simulink model "AC_DER_basic_model"  (R2021b)
settings: Solver=ode3  StartTime=0.0  StopTime=0.1  FixedStep=Ts  MaxStep=0.001  RelTol=1e-3  EnableMultiTasking=on
PostLoadFcn:
  | Ts=100e-6;
InitFcn:
  | Ts=100e-6;
libraries: fl_lib x5, nesl_utility x5, opal_lib x3, rtlab x2, ee_lib x2, spsRMSLib x2
Description:
  | Full-Wave Bridge Rectifier
  | 
  | This is a model of a power supply that converts 120 volts AC to 12  volts DC. The
  | transformer has a turns ratio of 14, stepping the supply down to 8.6 volts rms, i.e.
  | 8.6*sqrt(2) = 12 volts pk-pk. The full-wave bridge rectifier plus capacitor combination
  | then converts this to DC. The resistor represents a typical load.
  | 
  | The model can be used to size the capacitor required for a specified load.  For a
  | given size of capacitor, as the load resistance is increased, the ripple on the DC
  | voltage increases. The model can also be used to drive an application circuit in
  | order to assess the effect of the ripple.
  | 
  | 
  | Copyright 2008 The MathWorks(TM), Inc.
settings Model: Creator=rhyde  LastModifiedBy=fghow
settings SolverCC: AlgebraicLoopSolver=TrustRegion
settings DataIOCC: LimitDataPoints=on  SaveFormat=Array  SignalLoggingSaveFormat=ModelDataLogs  SaveOutput=off  SignalLogging=off  SaveTime=off  ReturnWorkspaceOutputs=off
settings OptimizationCC: BlockReduction=off  OptimizeBlockIOStorage=off  BufferReuse=off  ExpressionFolding=off  ExpressionDepthLimit=2147483647  LocalBlockOutputs=off  InitFltsAndDblsToZero=on  LifeSpan=inf
settings DebuggingCC: SaveWithParameterizedLinksMsg=none  UnderspecifiedInitializationDetection=Classic  MergeDetectMultiDrivingBlocksExec=none  SignalResolutionControl=TryResolveAllWithWarning  SolverPrmCheckMsg=warning  FcnCallInpInsideContextMsg=warning  StateNameClashWarn=warning  SFUnexpectedBacktrackingDiag=warning  SFNoUnconditionalDefaultTransitionDiag=warning  SFExecutionAtInitializationDiag=none  SFMachineParentedDataDiag=warning  ArithmeticOperatorsInVariantConditions=warning
settings HardwareCC: ProdBitPerPointer=32  ProdBitPerSizeT=32  ProdBitPerPtrDiffT=32  ProdLargestAtomicFloat=None  ProdIntDivRoundTo=Undefined  ProdEndianess=Unspecified  ProdWordSize=32  ProdHWDeviceType=32-bit Generic
settings ModelReferenceCC: PropagateSignalLabelsOutOfModel=off
settings SFSimCC: SimUseLocalCustomCode=off  CustomCodeUndefinedFunction=UseInterfaceOnly
settings RTWCC: RTWUseLocalCustomCode=off
settings CodeAppCC: StateflowObjectComments=on
settings GRTTargetCC: TargetFcnLib=ansi_tfl_tmw.mat  TargetLangStandard=C89/C90 (ANSI)  CombineOutputUpdateFcns=off  GRTInterface=on
settings ConfigComp: CovMetricSettings=dw  CovSaveCumulativeToWorkspaceVar=on  CovSaveSingleToWorkspaceVar=on  CovExternalEMLEnable=off
settings SimscapeCC: SimscapeNormalizeSystem=off

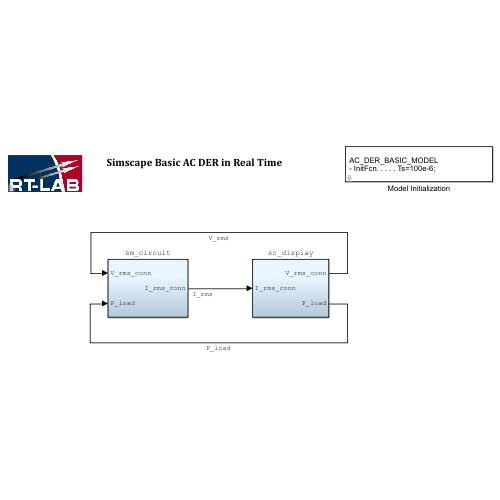
[thumbnail: Simulink's stored preview of the top-level diagram]
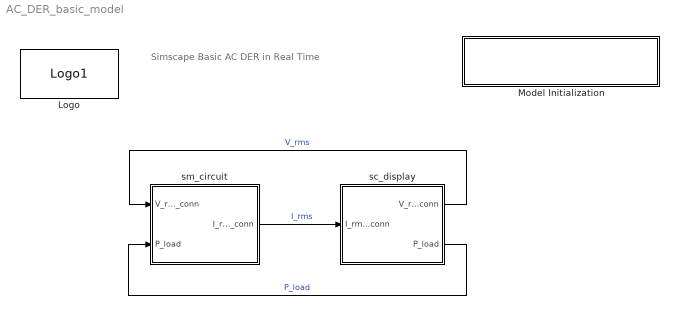
== system AC_DER_basic_model ==
  note: Simscape Basic AC DER in Real Time
  Logo : opal_lib/Logo1  vide=[]
  Model Initialization : Subsystem  mask(Model Functions){InitFcnX=Ts=100e-6;, prel=off, posl=on, inif=on, strf=off}
      mask prompts: InitFcnX "Initialisation"; prel "Preload Function"; posl "PostLoad Function"; inif "InitFcn"; strf "StartFcn"
      mask init:
      | currentBlock = gcb;
      | root = bdroot(currentBlock);
      | 
      | if ~strcmp(get_param(root,'BlockDiagramType'),'library')
      |     if prel==1
      |         set_param(root, 'PreLoadFcn', InitFcnX);
      |     else
      |         set_param(root, 'PreLoadFcn', '');
      |     end
      |     if inif==1
      |         set_param(root, 'InitFcn', InitFcnX);
      |     else
      |         set_param(root, 'InitFcn', '');
      |     end
      |     if strf==1
      |         set_param(root, 'StartFcn', InitFcnX);
      |     else
      |         set_param(root, 'StartFcn', '');
      |     end
      |     if posl==1
      |         set_param(root, 'PostLoadFcn', InitFcnX);
      |     else
      |         set_param(root, 'PostLoadFcn', '');
      |     end
      | end
      | 
      | pos = get_param(currentBlock, 'Position');
      | width = pos(3) - pos(1); height = pos(4) - pos(2);
      | txt = [ upper(root) '\n' '- InitFcn. . . . . '  get_param(root, 'InitFcn') ];
      settings: CopyFcn=set_param(gcb,'LinkStatus','none')
      mask Display: text(5, height*0.5, txt, 'horizontalAlignment', 'left', 'verticalAlignment', 'middle') ;
  sc_display : Subsystem
  sm_circuit : Subsystem
  wires:
  sm_circuit/1(I_rms_conn) -> sc_display/1(I_rms_conn)  "I_rms"
  sc_display/1(V_rms_conn) -> sm_circuit/1(V_rms_conn)  "V_rms"
  sc_display/2(P_load) -> sm_circuit/2(P_load)  "P_load"

== system AC_DER_basic_model/Model Initialization ==

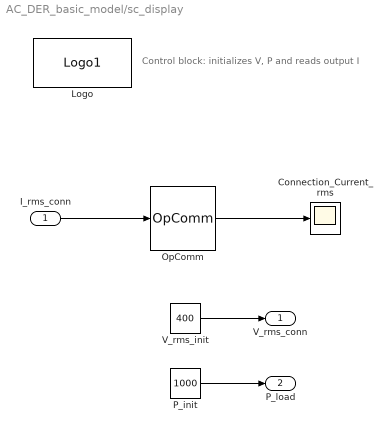
== system AC_DER_basic_model/sc_display ==
  note: Control block: initializes V, P and reads output I
  I_rms_conn : Inport
  Connection_Current_rms : Scope
  Logo : opal_lib/Logo1  vide=[]
  OpComm : rtlab/OpComm  nbport=1  groupe_acq=1  subsys_rate=0  st=0  Synchronization=on  Interpolation=on  Threshold=1.0  Missed_Data=off  Sim_Time=off  Samples=off  dynSigOut=off  from_console=0  warning_done=off  writeOpCommFile=off  Offset=off
      settings: SourceProductName=RT-LAB
  P_init : Constant  Value=1000
  V_rms_init : Constant  Value=400
  V_rms_conn : Outport
  P_load : Outport  Port=2
  wires:
  I_rms_conn/1 -> OpComm/1
  OpComm/1 -> Connection_Current_rms/1
  V_rms_init/1 -> V_rms_conn/1
  P_init/1 -> P_load/1

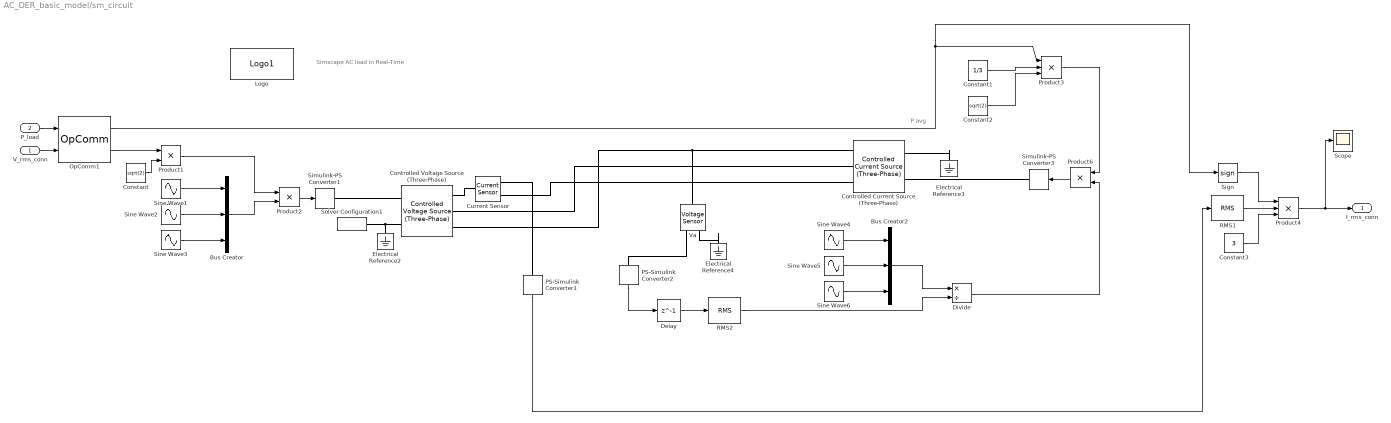
== system AC_DER_basic_model/sm_circuit ==
  note: Simscape AC load in Real-Time
  note: P avg
  V_rms_conn : Inport
  P_load : Inport  Port=2
  Bus Creator : BusCreator  Inputs=3
  Bus Creator2 : BusCreator  Inputs=3
  Constant : Constant  Value=sqrt(2)
  Constant1 : Constant  Value=1/3
  Constant2 : Constant  Value=sqrt(2)
  Constant3 : Constant  Value=3
  Controlled Current Source (Three-Phase) : ee_lib/Sources/Controlled Current Source (Three-Phase)
      settings: SourceProductBaseCode=PS  InternalSimscapePortConfiguration="{\"Bottom\":[],\"Left\":[{\"id\":\"S\",\"label\":\"S\",\"type\":\"input\"},{\"id\":\"n\",\"label\":\"n\",\"type\":\"foundation.electrical.electrical\"}],\"Right\":[{\"id\":\"a\",\"label\":\"a\",\"type\":\"foundation.electrical.electrical\"},{\"id\":\"b\",\"label\":\"b\",\"type\":\"foundation.electrical.electrical\"},{\"id\":\"c\",\"label\":\"c\",\"type\":\"foundation.electrical.electrical\"}],\"Top\":[]}"
  Controlled Voltage Source (Three-Phase) : ee_lib/Sources/Controlled Voltage Source (Three-Phase)
      settings: SourceProductBaseCode=PS  InternalSimscapePortConfiguration="{\"Bottom\":[],\"Left\":[{\"id\":\"S\",\"label\":\"S\",\"type\":\"input\"},{\"id\":\"n\",\"label\":\"n\",\"type\":\"foundation.electrical.electrical\"}],\"Right\":[{\"id\":\"a\",\"label\":\"a\",\"type\":\"foundation.electrical.electrical\"},{\"id\":\"b\",\"label\":\"b\",\"type\":\"foundation.electrical.electrical\"},{\"id\":\"c\",\"label\":\"c\",\"type\":\"foundation.electrical.electrical\"}],\"Top\":[]}"
  Current Sensor : fl_lib/Electrical/Electrical Sensors/Current Sensor
  Delay : Delay  DelayLength=1  InitialCondition=0
  Divide : Product  Inputs=*/
  Electrical Reference2 : fl_lib/Electrical/Electrical Elements/Electrical Reference
  Electrical Reference3 : fl_lib/Electrical/Electrical Elements/Electrical Reference
  Electrical Reference4 : fl_lib/Electrical/Electrical Elements/Electrical Reference
  Logo : opal_lib/Logo1  vide=[]
  OpComm1 : rtlab/OpComm  nbport=2  groupe_acq=1  subsys_rate=0  st=0  Synchronization=on  Interpolation=on  Threshold=1.0  Missed_Data=off  Sim_Time=off  Samples=off  dynSigOut=off  from_console=1  warning_done=off  writeOpCommFile=off  Offset=off
      settings: SourceProductName=RT-LAB
  PS-Simulink Converter1 : nesl_utility/PS-Simulink Converter  PhysicalDomain=network_engine_domain  SubClassName=ps_output  LeftPortType=input  RightPortType=output  PseudoPeriodic=off  Frequencies=[]  Unit=1  AffineConversion=off
      settings: SourceProductBaseCode=PW,SS
  PS-Simulink Converter2 : nesl_utility/PS-Simulink Converter  PhysicalDomain=network_engine_domain  SubClassName=ps_output  LeftPortType=input  RightPortType=output  PseudoPeriodic=off  Frequencies=[]  Unit=1  AffineConversion=off
      settings: SourceProductBaseCode=PW,SS
  Product1 : Product
  Product2 : Product
  Product3 : Product  Inputs=3
  Product4 : Product  Inputs=3
  Product6 : Product
  RMS1 : spsRMSLib/RMS  TrueRMS=on  Freq=50  RMSInit=1000/(400*3)  Ts=0
  RMS2 : spsRMSLib/RMS  TrueRMS=on  Freq=50  RMSInit=400  Ts=0
  Scope : Scope
  Sign : Signum
  Simulink-PS Converter1 : nesl_utility/Simulink-PS Converter  PhysicalDomain=network_engine_domain  SubClassName=ps_input  LeftPortType=input  RightPortType=output  PseudoPeriodic=off  Frequencies=[]  NoiseDistribution=none  NoiseParameters=[]  Unit=1  AffineConversion=off  FilteringAndDerivatives=filter  SimscapeFilterOrder=1  InputFilterTimeConstant=.001  UdotUserProvided=0
      settings: SourceProductBaseCode=PW,SS
  Simulink-PS Converter3 : nesl_utility/Simulink-PS Converter  PhysicalDomain=network_engine_domain  SubClassName=ps_input  LeftPortType=input  RightPortType=output  PseudoPeriodic=off  Frequencies=[]  NoiseDistribution=none  NoiseParameters=[]  Unit=1  AffineConversion=off  FilteringAndDerivatives=zero  SimscapeFilterOrder=1  InputFilterTimeConstant=.001  UdotUserProvided=0
      settings: SourceProductBaseCode=PW,SS
  Sine Wave1 : Sin  Frequency=2*pi*50  SampleTime=0
  Sine Wave2 : Sin  Frequency=2*pi*50  Phase=-2*pi/3  SampleTime=0
  Sine Wave3 : Sin  Frequency=2*pi*50  Phase=2*pi/3  SampleTime=0
  Sine Wave4 : Sin  Frequency=2*pi*50  SampleTime=0
  Sine Wave5 : Sin  Frequency=2*pi*50  Phase=-2*pi/3  SampleTime=0
  Sine Wave6 : Sin  Frequency=2*pi*50  Phase=2*pi/3  SampleTime=0
  Solver Configuration1 : nesl_utility/Solver Configuration  PhysicalDomain=network_engine_domain  SubClassName=solver  LeftPortType=input  RightPortType=generic  Tones=[]  Harmonics=[]  SimulateNoise=off  Profile=off  UseLocalSampling=off  EnableSwitchedLinearOptims=on  FrequencyDomain=off  UseCCode=off  RelTol=0.001  AbsTol=1e-06  MinStep=1e-09  ToWorkspace=off  RevertToSquareIcSolve=off  NumHomotopyIterations=100  PhasorMode=off  PhasorModeNumHarmonics=1  DoDC=off  ResidualTolerance=1e-9  UseLocalSolver=off  LocalSolverChoice=NE_BACKWARD_EULER_ADVANCER  LocalSolverSampleTime=.001  DoFixedCost=off  MaxNonlinIter=12  MaxModeIter=2  ComputeImpulses=off  ImpulseIterations=2  LinearAlgebra=Sparse  EquationFormulation=NE_TIME_EF  DelaysMemoryBudget=1024  AutomaticFiltering=on  FilteringTimeConstant=0.001  PartitionStorageMethod=AS_NEEDED  PartitionMemoryBudget=1024  PartitionMethod=FAST
      settings: SourceProductBaseCode=PW,SS
  Va : fl_lib/Electrical/Electrical Sensors/Voltage Sensor
  I_rms_conn : Outport
  wires:
  P_load/1 -> OpComm1/1
  V_rms_conn/1 -> OpComm1/2
  OpComm1/1 -> Product3/1, Sign/1
  Constant/1 -> Product1/2
  Product2/1 -> Simulink-PS Converter1/1
  Product1/1 -> Product2/1
  Sine Wave1/1 -> Bus Creator/1
  Sine Wave2/1 -> Bus Creator/2
  Sine Wave3/1 -> Bus Creator/3
  Bus Creator/1 -> Product2/2
  Constant1/1 -> Product3/2
  Product6/1 -> Simulink-PS Converter3/1
  Product3/1 -> Product6/1
  Sine Wave5/1 -> Bus Creator2/2
  Sine Wave6/1 -> Bus Creator2/3
  Sine Wave4/1 -> Bus Creator2/1
  PS-Simulink Converter2/1 -> Delay/1
  Sign/1 -> Product4/1
  PS-Simulink Converter1/1 -> RMS1/1
  RMS1/1 -> Product4/2
  Product4/1 -> Scope/1, I_rms_conn/1
  OpComm1/2 -> Product1/1
  Constant2/1 -> Product3/3
  Bus Creator2/1 -> Divide/1
  RMS2/1 -> Divide/2
  Constant3/1 -> Product4/3
  Divide/1 -> Product6/2
  Delay/1 -> RMS2/1
  connections:
  Electrical Reference2/LConn1 -- Solver Configuration1/RConn1 -- Controlled Voltage Source (Three-Phase)/LConn2
  Controlled Current Source (Three-Phase)/RConn2 -- Controlled Voltage Source (Three-Phase)/RConn2
  Controlled Current Source (Three-Phase)/RConn3 -- Va/LConn1 -- Controlled Voltage Source (Three-Phase)/RConn3
  Controlled Current Source (Three-Phase)/RConn1 -- Current Sensor/RConn2
  Current Sensor/LConn1 -- Controlled Voltage Source (Three-Phase)/RConn1
  PS-Simulink Converter1/LConn1 -- Current Sensor/RConn1
  Simulink-PS Converter1/RConn1 -- Controlled Voltage Source (Three-Phase)/LConn1
  Electrical Reference3/LConn1 -- Controlled Current Source (Three-Phase)/LConn2
  Va/RConn1 -- PS-Simulink Converter2/LConn1
  Simulink-PS Converter3/RConn1 -- Controlled Current Source (Three-Phase)/LConn1
  Electrical Reference4/LConn1 -- Va/RConn2
